simulink model "TST_AccPed_DrvDemDes"  (R2016b)
settings: Solver=FixedStepDiscrete  StartTime=0.0  StopTime=simTime  FixedStep=sampleTime  RelTol=1e-3
values from neighbouring files (symbols this model uses):
  testCase = 1    [initTST_AccPed_DrvDemDes_001.m]    (also in initTST_AccPed_DrvDemDes_002.m = 2; initTST_AccPed_DrvDemDes_003.m = 3; initTST_AccPed_DrvDemDes_004.m = 4; initTST_AccPed_DrvDemDes_005.m = 5)
libraries: simulink x61, UnitTest_Lib x54
(part 1 of 2)
settings Model: Creator=zhengjinyan  LastModifiedBy=zhengjinyan
settings DebuggingCC: SignalRangeChecking=error

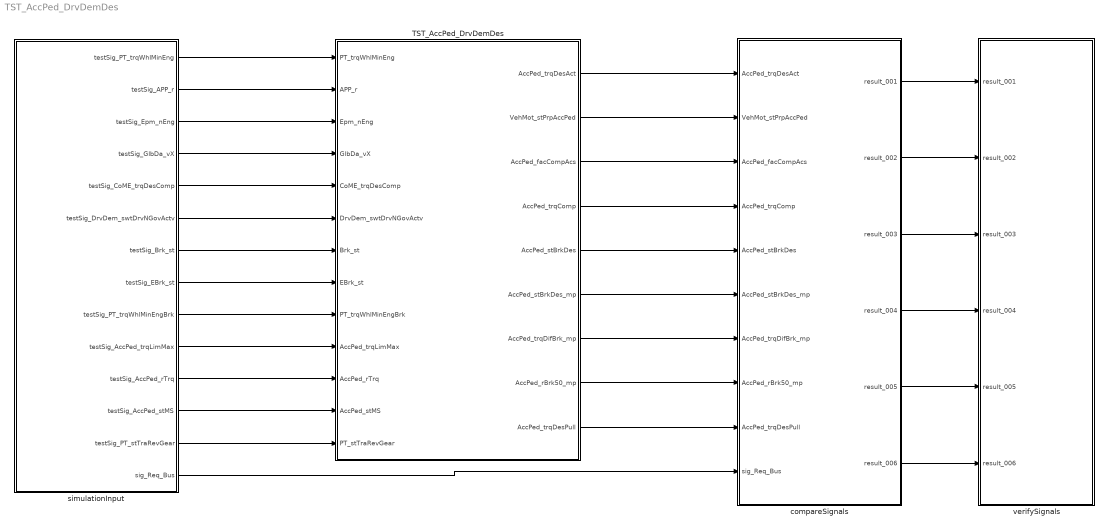
== system TST_AccPed_DrvDemDes ==
  TST_AccPed_DrvDemDes : Subsystem
  compareSignals : Subsystem
  simulationInput : Subsystem
  verifySignals : Subsystem
  wires:
  simulationInput/1(testSig_PT_trqWhlMinEng) -> TST_AccPed_DrvDemDes/1(PT_trqWhlMinEng)
  simulationInput/2(testSig_APP_r) -> TST_AccPed_DrvDemDes/2(APP_r)
  simulationInput/3(testSig_Epm_nEng) -> TST_AccPed_DrvDemDes/3(Epm_nEng)
  simulationInput/4(testSig_GlbDa_vX) -> TST_AccPed_DrvDemDes/4(GlbDa_vX)
  simulationInput/5(testSig_CoME_trqDesComp) -> TST_AccPed_DrvDemDes/5(CoME_trqDesComp)
  simulationInput/6(testSig_DrvDem_swtDrvNGovActv) -> TST_AccPed_DrvDemDes/6(DrvDem_swtDrvNGovActv)
  simulationInput/7(testSig_Brk_st) -> TST_AccPed_DrvDemDes/7(Brk_st)
  simulationInput/8(testSig_EBrk_st) -> TST_AccPed_DrvDemDes/8(EBrk_st)
  simulationInput/9(testSig_PT_trqWhlMinEngBrk) -> TST_AccPed_DrvDemDes/9(PT_trqWhlMinEngBrk)
  simulationInput/10(testSig_AccPed_trqLimMax) -> TST_AccPed_DrvDemDes/10(AccPed_trqLimMax)
  simulationInput/11(testSig_AccPed_rTrq) -> TST_AccPed_DrvDemDes/11(AccPed_rTrq)
  simulationInput/12(testSig_AccPed_stMS) -> TST_AccPed_DrvDemDes/12(AccPed_stMS)
  simulationInput/13(testSig_PT_stTraRevGear) -> TST_AccPed_DrvDemDes/13(PT_stTraRevGear)
  TST_AccPed_DrvDemDes/1(AccPed_trqDesAct) -> compareSignals/1(AccPed_trqDesAct)
  TST_AccPed_DrvDemDes/2(VehMot_stPrpAccPed) -> compareSignals/2(VehMot_stPrpAccPed)
  TST_AccPed_DrvDemDes/3(AccPed_facCompAcs) -> compareSignals/3(AccPed_facCompAcs)
  TST_AccPed_DrvDemDes/4(AccPed_trqComp) -> compareSignals/4(AccPed_trqComp)
  TST_AccPed_DrvDemDes/5(AccPed_stBrkDes) -> compareSignals/5(AccPed_stBrkDes)
  TST_AccPed_DrvDemDes/6(AccPed_stBrkDes_mp) -> compareSignals/6(AccPed_stBrkDes_mp)
  TST_AccPed_DrvDemDes/7(AccPed_trqDifBrk_mp) -> compareSignals/7(AccPed_trqDifBrk_mp)
  TST_AccPed_DrvDemDes/8(AccPed_rBrk50_mp) -> compareSignals/8(AccPed_rBrk50_mp)
  TST_AccPed_DrvDemDes/9(AccPed_trqDesPull) -> compareSignals/9(AccPed_trqDesPull)
  simulationInput/14(sig_Req_Bus) -> compareSignals/10(sig_Req_Bus)
  compareSignals/1(result_001) -> verifySignals/1(result_001)
  compareSignals/2(result_002) -> verifySignals/2(result_002)
  compareSignals/3(result_003) -> verifySignals/3(result_003)
  compareSignals/4(result_004) -> verifySignals/4(result_004)
  compareSignals/5(result_005) -> verifySignals/5(result_005)
  compareSignals/6(result_006) -> verifySignals/6(result_006)

== system TST_AccPed_DrvDemDes/TST_AccPed_DrvDemDes ==
  PT_trqWhlMinEng : Inport
  APP_r : Inport  Port=2
  Epm_nEng : Inport  Port=3
  GlbDa_vX : Inport  Port=4
  CoME_trqDesComp : Inport  Port=5
  DrvDem_swtDrvNGovActv : Inport  Port=6
  Brk_st : Inport  Port=7
  EBrk_st : Inport  Port=8
  PT_trqWhlMinEngBrk : Inport  Port=9
  AccPed_trqLimMax : Inport  Port=10
  AccPed_rTrq : Inport  Port=11
  AccPed_stMS : Inport  Port=12
  PT_stTraRevGear : Inport  Port=13
  AccPed_DrvDemDes : ModelReference  ModelNameDialog=AccPed_DrvDemDes  SimulationMode=Normal  ModelReferenceVersion=1.64  TriggerPortName=function  TriggerPortTriggerType=function-call  TriggerPortStatesWhenEnabling=held
  Function_Call : simulink/Ports & Subsystems/Function-Call Generator  sample_time=sampleTime  numberOfIterations=1
  AccPed_trqDesAct : Outport
  VehMot_stPrpAccPed : Outport  Port=2
  AccPed_facCompAcs : Outport  Port=3
  AccPed_trqComp : Outport  Port=4
  AccPed_stBrkDes : Outport  Port=5
  AccPed_stBrkDes_mp : Outport  Port=6
  AccPed_trqDifBrk_mp : Outport  Port=7
  AccPed_rBrk50_mp : Outport  Port=8
  AccPed_trqDesPull : Outport  Port=9
  wires:
  Function_Call/1 -> AccPed_DrvDemDes/Trigger
  PT_trqWhlMinEng/1 -> AccPed_DrvDemDes/1
  APP_r/1 -> AccPed_DrvDemDes/2
  Epm_nEng/1 -> AccPed_DrvDemDes/3
  GlbDa_vX/1 -> AccPed_DrvDemDes/4
  CoME_trqDesComp/1 -> AccPed_DrvDemDes/5
  DrvDem_swtDrvNGovActv/1 -> AccPed_DrvDemDes/6
  Brk_st/1 -> AccPed_DrvDemDes/7
  EBrk_st/1 -> AccPed_DrvDemDes/8
  PT_trqWhlMinEngBrk/1 -> AccPed_DrvDemDes/9
  AccPed_trqLimMax/1 -> AccPed_DrvDemDes/10
  AccPed_rTrq/1 -> AccPed_DrvDemDes/11
  AccPed_stMS/1 -> AccPed_DrvDemDes/12
  PT_stTraRevGear/1 -> AccPed_DrvDemDes/13
  AccPed_DrvDemDes/1 -> AccPed_trqDesAct/1
  AccPed_DrvDemDes/2 -> VehMot_stPrpAccPed/1
  AccPed_DrvDemDes/3 -> AccPed_facCompAcs/1
  AccPed_DrvDemDes/4 -> AccPed_trqComp/1
  AccPed_DrvDemDes/5 -> AccPed_stBrkDes/1
  AccPed_DrvDemDes/6 -> AccPed_stBrkDes_mp/1
  AccPed_DrvDemDes/7 -> AccPed_trqDifBrk_mp/1
  AccPed_DrvDemDes/8 -> AccPed_rBrk50_mp/1
  AccPed_DrvDemDes/9 -> AccPed_trqDesPull/1

== system TST_AccPed_DrvDemDes/compareSignals ==
  AccPed_trqDesAct : Inport
  VehMot_stPrpAccPed : Inport  Port=2
  AccPed_facCompAcs : Inport  Port=3
  AccPed_trqComp : Inport  Port=4
  AccPed_stBrkDes : Inport  Port=5
  AccPed_stBrkDes_mp : Inport  Port=6
  AccPed_trqDifBrk_mp : Inport  Port=7
  AccPed_rBrk50_mp : Inport  Port=8
  AccPed_trqDesPull : Inport  Port=9
  sig_Req_Bus : Inport  Port=10
  BC : BusCreator  Inputs=9
  CTC_001 : simulink/Logic and Bit Operations/Compare To Constant  relop===  const=1  OutDataTypeStr=boolean
  CTC_002 : simulink/Logic and Bit Operations/Compare To Constant  relop===  const=2  OutDataTypeStr=boolean
  CTC_003 : simulink/Logic and Bit Operations/Compare To Constant  relop===  const=3  OutDataTypeStr=boolean
  CTC_004 : simulink/Logic and Bit Operations/Compare To Constant  relop===  const=4  OutDataTypeStr=boolean
  CTC_005 : simulink/Logic and Bit Operations/Compare To Constant  relop===  const=5  OutDataTypeStr=boolean
  CTC_006 : simulink/Logic and Bit Operations/Compare To Constant  relop===  const=6  OutDataTypeStr=boolean
  Requirement_001 : Subsystem
  Requirement_002 : Subsystem
  Requirement_003 : Subsystem
  Requirement_004 : Subsystem
  Requirement_005 : Subsystem
  Requirement_006 : Subsystem
  TC_001 : Constant  Value=testCase
  TC_002 : Constant  Value=testCase
  TC_003 : Constant  Value=testCase
  TC_004 : Constant  Value=testCase
  TC_005 : Constant  Value=testCase
  TC_006 : Constant  Value=testCase
  result_001 : Outport
  result_002 : Outport  Port=2
  result_003 : Outport  Port=3
  result_004 : Outport  Port=4
  result_005 : Outport  Port=5
  result_006 : Outport  Port=6
  wires:
  AccPed_trqDesAct/1 -> BC/1  "AccPed_trqDesAct"
  VehMot_stPrpAccPed/1 -> BC/2  "VehMot_stPrpAccPed"
  AccPed_facCompAcs/1 -> BC/3  "AccPed_facCompAcs"
  AccPed_trqComp/1 -> BC/4  "AccPed_trqComp"
  AccPed_stBrkDes/1 -> BC/5  "AccPed_stBrkDes"
  AccPed_stBrkDes_mp/1 -> BC/6  "AccPed_stBrkDes_mp"
  AccPed_trqDifBrk_mp/1 -> BC/7  "AccPed_trqDifBrk_mp"
  AccPed_rBrk50_mp/1 -> BC/8  "AccPed_rBrk50_mp"
  AccPed_trqDesPull/1 -> BC/9  "AccPed_trqDesPull"
  TC_001/1 -> CTC_001/1
  CTC_001/1 -> Requirement_001/Enable
  sig_Req_Bus/1 -> Requirement_001/2(sig_Req_Bus), Requirement_002/2(sig_Req_Bus), Requirement_003/2(sig_Req_Bus), Requirement_004/2(sig_Req_Bus), Requirement_005/2(sig_Req_Bus), Requirement_006/2(sig_Req_Bus)
  BC/1 -> Requirement_001/1(sig_Result_Bus), Requirement_002/1(sig_Result_Bus), Requirement_003/1(sig_Result_Bus), Requirement_004/1(sig_Result_Bus), Requirement_005/1(sig_Result_Bus), Requirement_006/1(sig_Result_Bus)
  Requirement_001/1(result) -> result_001/1
  TC_002/1 -> CTC_002/1
  CTC_002/1 -> Requirement_002/Enable
  Requirement_002/1(result) -> result_002/1
  TC_003/1 -> CTC_003/1
  CTC_003/1 -> Requirement_003/Enable
  Requirement_003/1(result) -> result_003/1
  TC_004/1 -> CTC_004/1
  CTC_004/1 -> Requirement_004/Enable
  Requirement_004/1(result) -> result_004/1
  TC_005/1 -> CTC_005/1
  CTC_005/1 -> Requirement_005/Enable
  Requirement_005/1(result) -> result_005/1
  TC_006/1 -> CTC_006/1
  CTC_006/1 -> Requirement_006/Enable
  Requirement_006/1(result) -> result_006/1

== system TST_AccPed_DrvDemDes/simulationInput ==
  BS : BusSelector  OutputSignals=testSig_PT_trqWhlMinEng,testSig_APP_r,testSig_Epm_nEng,testSig_GlbDa_vX,testSig_CoME_trqDesComp,testSig_DrvDem_swtDrvNGovActv,testSig_Brk_st,testSig_EBrk_st,testSig_PT_trqWhlMinEngBrk,testSig_AccPed_trqLimMax,testSig_AccPed_rTrq,testSig_AccPed_stMS,testSig_PT_stTraRevGear
  MPSw : MultiPortSwitch  Inputs=6  SaturateOnIntegerOverflow=on  InputSameDT=on
  TestCase : Constant  Value=testCase
  testSignals_R001 : Subsystem
  testSignals_R002 : Subsystem
  testSignals_R003 : Subsystem
  testSignals_R004 : Subsystem
  testSignals_R005 : Subsystem
  testSignals_R006 : Subsystem
  testSig_PT_trqWhlMinEng : Outport
  testSig_APP_r : Outport  Port=2
  testSig_Epm_nEng : Outport  Port=3
  testSig_GlbDa_vX : Outport  Port=4
  testSig_CoME_trqDesComp : Outport  Port=5
  testSig_DrvDem_swtDrvNGovActv : Outport  Port=6
  testSig_Brk_st : Outport  Port=7
  testSig_EBrk_st : Outport  Port=8
  testSig_PT_trqWhlMinEngBrk : Outport  Port=9
  testSig_AccPed_trqLimMax : Outport  Port=10
  testSig_AccPed_rTrq : Outport  Port=11
  testSig_AccPed_stMS : Outport  Port=12
  testSig_PT_stTraRevGear : Outport  Port=13
  sig_Req_Bus : Outport  Port=14
  wires:
  BS/1 -> testSig_PT_trqWhlMinEng/1  "<testSig_PT_trqWhlMinEng>"
  BS/2 -> testSig_APP_r/1  "<testSig_APP_r>"
  BS/3 -> testSig_Epm_nEng/1  "<testSig_Epm_nEng>"
  BS/4 -> testSig_GlbDa_vX/1  "<testSig_GlbDa_vX>"
  BS/5 -> testSig_CoME_trqDesComp/1  "<testSig_CoME_trqDesComp>"
  BS/6 -> testSig_DrvDem_swtDrvNGovActv/1  "<testSig_DrvDem_swtDrvNGovActv>"
  BS/7 -> testSig_Brk_st/1  "<testSig_Brk_st>"
  BS/8 -> testSig_EBrk_st/1  "<testSig_EBrk_st>"
  BS/9 -> testSig_PT_trqWhlMinEngBrk/1  "<testSig_PT_trqWhlMinEngBrk>"
  BS/10 -> testSig_AccPed_trqLimMax/1  "<testSig_AccPed_trqLimMax>"
  BS/11 -> testSig_AccPed_rTrq/1  "<testSig_AccPed_rTrq>"
  BS/12 -> testSig_AccPed_stMS/1  "<testSig_AccPed_stMS>"
  BS/13 -> testSig_PT_stTraRevGear/1  "<testSig_PT_stTraRevGear>"
  MPSw/1 -> BS/1, sig_Req_Bus/1
  TestCase/1 -> MPSw/1
  testSignals_R001/1(testSignals) -> MPSw/2
  testSignals_R002/1(testSignals) -> MPSw/3
  testSignals_R003/1(testSignals) -> MPSw/4
  testSignals_R004/1(testSignals) -> MPSw/5
  testSignals_R005/1(testSignals) -> MPSw/6
  testSignals_R006/1(testSignals) -> MPSw/7

== system TST_AccPed_DrvDemDes/verifySignals ==
  result_001 : Inport
  result_002 : Inport  Port=2
  result_003 : Inport  Port=3
  result_004 : Inport  Port=4
  result_005 : Inport  Port=5
  result_006 : Inport  Port=6
  Assertion_001 : Assertion  Enabled=off
  Assertion_002 : Assertion  Enabled=off
  Assertion_003 : Assertion  Enabled=off
  Assertion_004 : Assertion  Enabled=off
  Assertion_005 : Assertion  Enabled=off
  Assertion_006 : Assertion  Enabled=off
  wires:
  result_001/1 -> Assertion_001/1
  result_002/1 -> Assertion_002/1
  result_003/1 -> Assertion_003/1
  result_004/1 -> Assertion_004/1
  result_005/1 -> Assertion_005/1
  result_006/1 -> Assertion_006/1

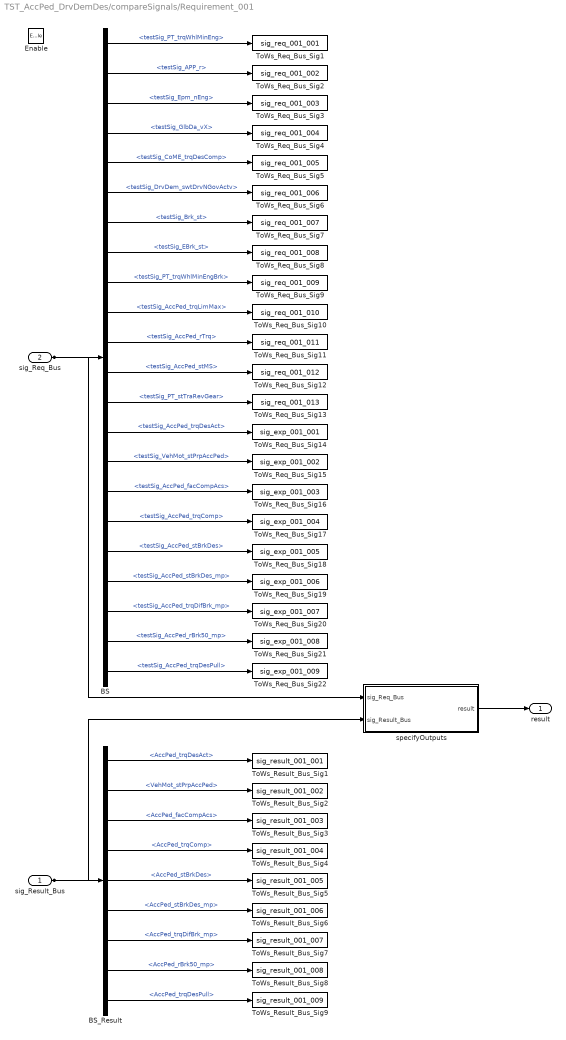
== system TST_AccPed_DrvDemDes/compareSignals/Requirement_001 ==
  sig_Result_Bus : Inport
  sig_Req_Bus : Inport  Port=2
  Enable : EnablePort
  BS : BusSelector  OutputSignals=testSig_PT_trqWhlMinEng,testSig_APP_r,testSig_Epm_nEng,testSig_GlbDa_vX,testSig_CoME_trqDesComp,testSig_DrvDem_swtDrvNGovActv,testSig_Brk_st,testSig_EBrk_st,testSig_PT_trqWhlMinEngBrk,testSig_AccPed_trqLimMax,testSig_AccPed_rTrq,testSig_AccPed_stMS,testSig_PT_stTraRevGear,testSig_AccPed_trqDesAct,testSig_VehMot_stPrpAccPed,testSig_AccPed_facCompAcs,testSig_AccPed_trqComp,testSig_AccPed_stBrkDes,testSig_AccPed_stBrkDes_mp,testSig_AccPed_trqDifBrk_mp,testSig_AccPed_rBrk50_mp,testSig_AccPed_trqDesPull
  BS_Result : BusSelector  OutputSignals=AccPed_trqDesAct,VehMot_stPrpAccPed,AccPed_facCompAcs,AccPed_trqComp,AccPed_stBrkDes,AccPed_stBrkDes_mp,AccPed_trqDifBrk_mp,AccPed_rBrk50_mp,AccPed_trqDesPull
  ToWs_Req_Bus_Sig1 : ToWorkspace  VariableName=sig_req_001_001  SaveFormat=Structure With Time
  ToWs_Req_Bus_Sig10 : ToWorkspace  VariableName=sig_req_001_010  SaveFormat=Structure With Time
  ToWs_Req_Bus_Sig11 : ToWorkspace  VariableName=sig_req_001_011  SaveFormat=Structure With Time
  ToWs_Req_Bus_Sig12 : ToWorkspace  VariableName=sig_req_001_012  SaveFormat=Structure With Time
  ToWs_Req_Bus_Sig13 : ToWorkspace  VariableName=sig_req_001_013  SaveFormat=Structure With Time
  ToWs_Req_Bus_Sig14 : ToWorkspace  VariableName=sig_exp_001_001  SaveFormat=Structure With Time
  ToWs_Req_Bus_Sig15 : ToWorkspace  VariableName=sig_exp_001_002  SaveFormat=Structure With Time
  ToWs_Req_Bus_Sig16 : ToWorkspace  VariableName=sig_exp_001_003  SaveFormat=Structure With Time
  ToWs_Req_Bus_Sig17 : ToWorkspace  VariableName=sig_exp_001_004  SaveFormat=Structure With Time
  ToWs_Req_Bus_Sig18 : ToWorkspace  VariableName=sig_exp_001_005  SaveFormat=Structure With Time
  ToWs_Req_Bus_Sig19 : ToWorkspace  VariableName=sig_exp_001_006  SaveFormat=Structure With Time
  ToWs_Req_Bus_Sig2 : ToWorkspace  VariableName=sig_req_001_002  SaveFormat=Structure With Time
  ToWs_Req_Bus_Sig20 : ToWorkspace  VariableName=sig_exp_001_007  SaveFormat=Structure With Time
  ToWs_Req_Bus_Sig21 : ToWorkspace  VariableName=sig_exp_001_008  SaveFormat=Structure With Time
  ToWs_Req_Bus_Sig22 : ToWorkspace  VariableName=sig_exp_001_009  SaveFormat=Structure With Time
  ToWs_Req_Bus_Sig3 : ToWorkspace  VariableName=sig_req_001_003  SaveFormat=Structure With Time
  ToWs_Req_Bus_Sig4 : ToWorkspace  VariableName=sig_req_001_004  SaveFormat=Structure With Time
  ToWs_Req_Bus_Sig5 : ToWorkspace  VariableName=sig_req_001_005  SaveFormat=Structure With Time
  ToWs_Req_Bus_Sig6 : ToWorkspace  VariableName=sig_req_001_006  SaveFormat=Structure With Time
  ToWs_Req_Bus_Sig7 : ToWorkspace  VariableName=sig_req_001_007  SaveFormat=Structure With Time
  ToWs_Req_Bus_Sig8 : ToWorkspace  VariableName=sig_req_001_008  SaveFormat=Structure With Time
  ToWs_Req_Bus_Sig9 : ToWorkspace  VariableName=sig_req_001_009  SaveFormat=Structure With Time
  ToWs_Result_Bus_Sig1 : ToWorkspace  VariableName=sig_result_001_001  SaveFormat=Structure With Time
  ToWs_Result_Bus_Sig2 : ToWorkspace  VariableName=sig_result_001_002  SaveFormat=Structure With Time
  ToWs_Result_Bus_Sig3 : ToWorkspace  VariableName=sig_result_001_003  SaveFormat=Structure With Time
  ToWs_Result_Bus_Sig4 : ToWorkspace  VariableName=sig_result_001_004  SaveFormat=Structure With Time
  ToWs_Result_Bus_Sig5 : ToWorkspace  VariableName=sig_result_001_005  SaveFormat=Structure With Time
  ToWs_Result_Bus_Sig6 : ToWorkspace  VariableName=sig_result_001_006  SaveFormat=Structure With Time
  ToWs_Result_Bus_Sig7 : ToWorkspace  VariableName=sig_result_001_007  SaveFormat=Structure With Time
  ToWs_Result_Bus_Sig8 : ToWorkspace  VariableName=sig_result_001_008  SaveFormat=Structure With Time
  ToWs_Result_Bus_Sig9 : ToWorkspace  VariableName=sig_result_001_009  SaveFormat=Structure With Time
  specifyOutputs : Subsystem
  result : Outport
  wires:
  sig_Req_Bus/1 -> BS/1, specifyOutputs/1(sig_Req_Bus)
  BS/1 -> ToWs_Req_Bus_Sig1/1  "<testSig_PT_trqWhlMinEng>"
  BS/2 -> ToWs_Req_Bus_Sig2/1  "<testSig_APP_r>"
  BS/3 -> ToWs_Req_Bus_Sig3/1  "<testSig_Epm_nEng>"
  BS/4 -> ToWs_Req_Bus_Sig4/1  "<testSig_GlbDa_vX>"
  BS/5 -> ToWs_Req_Bus_Sig5/1  "<testSig_CoME_trqDesComp>"
  BS/6 -> ToWs_Req_Bus_Sig6/1  "<testSig_DrvDem_swtDrvNGovActv>"
  BS/7 -> ToWs_Req_Bus_Sig7/1  "<testSig_Brk_st>"
  BS/8 -> ToWs_Req_Bus_Sig8/1  "<testSig_EBrk_st>"
  BS/9 -> ToWs_Req_Bus_Sig9/1  "<testSig_PT_trqWhlMinEngBrk>"
  BS/10 -> ToWs_Req_Bus_Sig10/1  "<testSig_AccPed_trqLimMax>"
  BS/11 -> ToWs_Req_Bus_Sig11/1  "<testSig_AccPed_rTrq>"
  BS/12 -> ToWs_Req_Bus_Sig12/1  "<testSig_AccPed_stMS>"
  BS/13 -> ToWs_Req_Bus_Sig13/1  "<testSig_PT_stTraRevGear>"
  BS/14 -> ToWs_Req_Bus_Sig14/1  "<testSig_AccPed_trqDesAct>"
  BS/15 -> ToWs_Req_Bus_Sig15/1  "<testSig_VehMot_stPrpAccPed>"
  BS/16 -> ToWs_Req_Bus_Sig16/1  "<testSig_AccPed_facCompAcs>"
  BS/17 -> ToWs_Req_Bus_Sig17/1  "<testSig_AccPed_trqComp>"
  BS/18 -> ToWs_Req_Bus_Sig18/1  "<testSig_AccPed_stBrkDes>"
  BS/19 -> ToWs_Req_Bus_Sig19/1  "<testSig_AccPed_stBrkDes_mp>"
  BS/20 -> ToWs_Req_Bus_Sig20/1  "<testSig_AccPed_trqDifBrk_mp>"
  BS/21 -> ToWs_Req_Bus_Sig21/1  "<testSig_AccPed_rBrk50_mp>"
  BS/22 -> ToWs_Req_Bus_Sig22/1  "<testSig_AccPed_trqDesPull>"
  sig_Result_Bus/1 -> BS_Result/1, specifyOutputs/2(sig_Result_Bus)
  BS_Result/1 -> ToWs_Result_Bus_Sig1/1  "<AccPed_trqDesAct>"
  BS_Result/2 -> ToWs_Result_Bus_Sig2/1  "<VehMot_stPrpAccPed>"
  BS_Result/3 -> ToWs_Result_Bus_Sig3/1  "<AccPed_facCompAcs>"
  BS_Result/4 -> ToWs_Result_Bus_Sig4/1  "<AccPed_trqComp>"
  BS_Result/5 -> ToWs_Result_Bus_Sig5/1  "<AccPed_stBrkDes>"
  BS_Result/6 -> ToWs_Result_Bus_Sig6/1  "<AccPed_stBrkDes_mp>"
  BS_Result/7 -> ToWs_Result_Bus_Sig7/1  "<AccPed_trqDifBrk_mp>"
  BS_Result/8 -> ToWs_Result_Bus_Sig8/1  "<AccPed_rBrk50_mp>"
  BS_Result/9 -> ToWs_Result_Bus_Sig9/1  "<AccPed_trqDesPull>"
  specifyOutputs/1(result) -> result/1

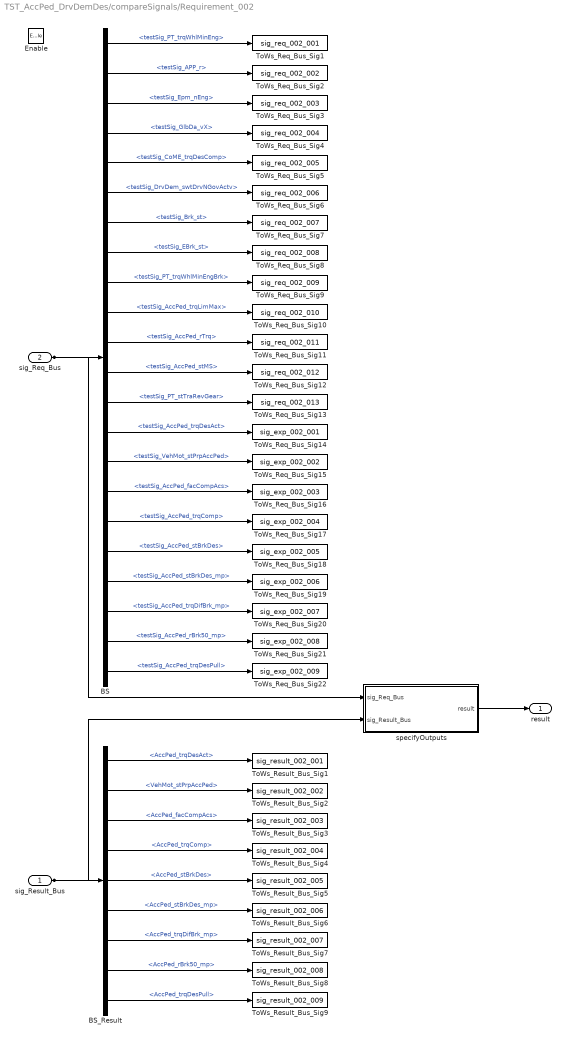
== system TST_AccPed_DrvDemDes/compareSignals/Requirement_002 ==
  sig_Result_Bus : Inport
  sig_Req_Bus : Inport  Port=2
  Enable : EnablePort
  BS : BusSelector  OutputSignals=testSig_PT_trqWhlMinEng,testSig_APP_r,testSig_Epm_nEng,testSig_GlbDa_vX,testSig_CoME_trqDesComp,testSig_DrvDem_swtDrvNGovActv,testSig_Brk_st,testSig_EBrk_st,testSig_PT_trqWhlMinEngBrk,testSig_AccPed_trqLimMax,testSig_AccPed_rTrq,testSig_AccPed_stMS,testSig_PT_stTraRevGear,testSig_AccPed_trqDesAct,testSig_VehMot_stPrpAccPed,testSig_AccPed_facCompAcs,testSig_AccPed_trqComp,testSig_AccPed_stBrkDes,testSig_AccPed_stBrkDes_mp,testSig_AccPed_trqDifBrk_mp,testSig_AccPed_rBrk50_mp,testSig_AccPed_trqDesPull
  BS_Result : BusSelector  OutputSignals=AccPed_trqDesAct,VehMot_stPrpAccPed,AccPed_facCompAcs,AccPed_trqComp,AccPed_stBrkDes,AccPed_stBrkDes_mp,AccPed_trqDifBrk_mp,AccPed_rBrk50_mp,AccPed_trqDesPull
  ToWs_Req_Bus_Sig1 : ToWorkspace  VariableName=sig_req_002_001  SaveFormat=Structure With Time
  ToWs_Req_Bus_Sig10 : ToWorkspace  VariableName=sig_req_002_010  SaveFormat=Structure With Time
  ToWs_Req_Bus_Sig11 : ToWorkspace  VariableName=sig_req_002_011  SaveFormat=Structure With Time
  ToWs_Req_Bus_Sig12 : ToWorkspace  VariableName=sig_req_002_012  SaveFormat=Structure With Time
  ToWs_Req_Bus_Sig13 : ToWorkspace  VariableName=sig_req_002_013  SaveFormat=Structure With Time
  ToWs_Req_Bus_Sig14 : ToWorkspace  VariableName=sig_exp_002_001  SaveFormat=Structure With Time
  ToWs_Req_Bus_Sig15 : ToWorkspace  VariableName=sig_exp_002_002  SaveFormat=Structure With Time
  ToWs_Req_Bus_Sig16 : ToWorkspace  VariableName=sig_exp_002_003  SaveFormat=Structure With Time
  ToWs_Req_Bus_Sig17 : ToWorkspace  VariableName=sig_exp_002_004  SaveFormat=Structure With Time
  ToWs_Req_Bus_Sig18 : ToWorkspace  VariableName=sig_exp_002_005  SaveFormat=Structure With Time
  ToWs_Req_Bus_Sig19 : ToWorkspace  VariableName=sig_exp_002_006  SaveFormat=Structure With Time
  ToWs_Req_Bus_Sig2 : ToWorkspace  VariableName=sig_req_002_002  SaveFormat=Structure With Time
  ToWs_Req_Bus_Sig20 : ToWorkspace  VariableName=sig_exp_002_007  SaveFormat=Structure With Time
  ToWs_Req_Bus_Sig21 : ToWorkspace  VariableName=sig_exp_002_008  SaveFormat=Structure With Time
  ToWs_Req_Bus_Sig22 : ToWorkspace  VariableName=sig_exp_002_009  SaveFormat=Structure With Time
  ToWs_Req_Bus_Sig3 : ToWorkspace  VariableName=sig_req_002_003  SaveFormat=Structure With Time
  ToWs_Req_Bus_Sig4 : ToWorkspace  VariableName=sig_req_002_004  SaveFormat=Structure With Time
  ToWs_Req_Bus_Sig5 : ToWorkspace  VariableName=sig_req_002_005  SaveFormat=Structure With Time
  ToWs_Req_Bus_Sig6 : ToWorkspace  VariableName=sig_req_002_006  SaveFormat=Structure With Time
  ToWs_Req_Bus_Sig7 : ToWorkspace  VariableName=sig_req_002_007  SaveFormat=Structure With Time
  ToWs_Req_Bus_Sig8 : ToWorkspace  VariableName=sig_req_002_008  SaveFormat=Structure With Time
  ToWs_Req_Bus_Sig9 : ToWorkspace  VariableName=sig_req_002_009  SaveFormat=Structure With Time
  ToWs_Result_Bus_Sig1 : ToWorkspace  VariableName=sig_result_002_001  SaveFormat=Structure With Time
  ToWs_Result_Bus_Sig2 : ToWorkspace  VariableName=sig_result_002_002  SaveFormat=Structure With Time
  ToWs_Result_Bus_Sig3 : ToWorkspace  VariableName=sig_result_002_003  SaveFormat=Structure With Time
  ToWs_Result_Bus_Sig4 : ToWorkspace  VariableName=sig_result_002_004  SaveFormat=Structure With Time
  ToWs_Result_Bus_Sig5 : ToWorkspace  VariableName=sig_result_002_005  SaveFormat=Structure With Time
  ToWs_Result_Bus_Sig6 : ToWorkspace  VariableName=sig_result_002_006  SaveFormat=Structure With Time
  ToWs_Result_Bus_Sig7 : ToWorkspace  VariableName=sig_result_002_007  SaveFormat=Structure With Time
  ToWs_Result_Bus_Sig8 : ToWorkspace  VariableName=sig_result_002_008  SaveFormat=Structure With Time
  ToWs_Result_Bus_Sig9 : ToWorkspace  VariableName=sig_result_002_009  SaveFormat=Structure With Time
  specifyOutputs : Subsystem
  result : Outport
  wires:
  sig_Req_Bus/1 -> BS/1, specifyOutputs/1(sig_Req_Bus)
  BS/1 -> ToWs_Req_Bus_Sig1/1  "<testSig_PT_trqWhlMinEng>"
  BS/2 -> ToWs_Req_Bus_Sig2/1  "<testSig_APP_r>"
  BS/3 -> ToWs_Req_Bus_Sig3/1  "<testSig_Epm_nEng>"
  BS/4 -> ToWs_Req_Bus_Sig4/1  "<testSig_GlbDa_vX>"
  BS/5 -> ToWs_Req_Bus_Sig5/1  "<testSig_CoME_trqDesComp>"
  BS/6 -> ToWs_Req_Bus_Sig6/1  "<testSig_DrvDem_swtDrvNGovActv>"
  BS/7 -> ToWs_Req_Bus_Sig7/1  "<testSig_Brk_st>"
  BS/8 -> ToWs_Req_Bus_Sig8/1  "<testSig_EBrk_st>"
  BS/9 -> ToWs_Req_Bus_Sig9/1  "<testSig_PT_trqWhlMinEngBrk>"
  BS/10 -> ToWs_Req_Bus_Sig10/1  "<testSig_AccPed_trqLimMax>"
  BS/11 -> ToWs_Req_Bus_Sig11/1  "<testSig_AccPed_rTrq>"
  BS/12 -> ToWs_Req_Bus_Sig12/1  "<testSig_AccPed_stMS>"
  BS/13 -> ToWs_Req_Bus_Sig13/1  "<testSig_PT_stTraRevGear>"
  BS/14 -> ToWs_Req_Bus_Sig14/1  "<testSig_AccPed_trqDesAct>"
  BS/15 -> ToWs_Req_Bus_Sig15/1  "<testSig_VehMot_stPrpAccPed>"
  BS/16 -> ToWs_Req_Bus_Sig16/1  "<testSig_AccPed_facCompAcs>"
  BS/17 -> ToWs_Req_Bus_Sig17/1  "<testSig_AccPed_trqComp>"
  BS/18 -> ToWs_Req_Bus_Sig18/1  "<testSig_AccPed_stBrkDes>"
  BS/19 -> ToWs_Req_Bus_Sig19/1  "<testSig_AccPed_stBrkDes_mp>"
  BS/20 -> ToWs_Req_Bus_Sig20/1  "<testSig_AccPed_trqDifBrk_mp>"
  BS/21 -> ToWs_Req_Bus_Sig21/1  "<testSig_AccPed_rBrk50_mp>"
  BS/22 -> ToWs_Req_Bus_Sig22/1  "<testSig_AccPed_trqDesPull>"
  sig_Result_Bus/1 -> BS_Result/1, specifyOutputs/2(sig_Result_Bus)
  BS_Result/1 -> ToWs_Result_Bus_Sig1/1  "<AccPed_trqDesAct>"
  BS_Result/2 -> ToWs_Result_Bus_Sig2/1  "<VehMot_stPrpAccPed>"
  BS_Result/3 -> ToWs_Result_Bus_Sig3/1  "<AccPed_facCompAcs>"
  BS_Result/4 -> ToWs_Result_Bus_Sig4/1  "<AccPed_trqComp>"
  BS_Result/5 -> ToWs_Result_Bus_Sig5/1  "<AccPed_stBrkDes>"
  BS_Result/6 -> ToWs_Result_Bus_Sig6/1  "<AccPed_stBrkDes_mp>"
  BS_Result/7 -> ToWs_Result_Bus_Sig7/1  "<AccPed_trqDifBrk_mp>"
  BS_Result/8 -> ToWs_Result_Bus_Sig8/1  "<AccPed_rBrk50_mp>"
  BS_Result/9 -> ToWs_Result_Bus_Sig9/1  "<AccPed_trqDesPull>"
  specifyOutputs/1(result) -> result/1

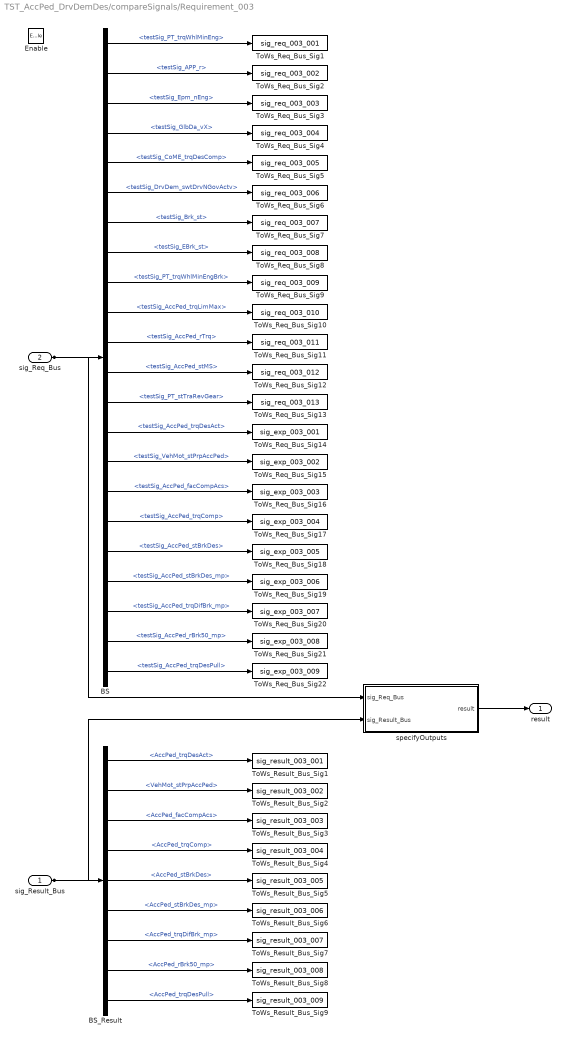
== system TST_AccPed_DrvDemDes/compareSignals/Requirement_003 ==
  sig_Result_Bus : Inport
  sig_Req_Bus : Inport  Port=2
  Enable : EnablePort
  BS : BusSelector  OutputSignals=testSig_PT_trqWhlMinEng,testSig_APP_r,testSig_Epm_nEng,testSig_GlbDa_vX,testSig_CoME_trqDesComp,testSig_DrvDem_swtDrvNGovActv,testSig_Brk_st,testSig_EBrk_st,testSig_PT_trqWhlMinEngBrk,testSig_AccPed_trqLimMax,testSig_AccPed_rTrq,testSig_AccPed_stMS,testSig_PT_stTraRevGear,testSig_AccPed_trqDesAct,testSig_VehMot_stPrpAccPed,testSig_AccPed_facCompAcs,testSig_AccPed_trqComp,testSig_AccPed_stBrkDes,testSig_AccPed_stBrkDes_mp,testSig_AccPed_trqDifBrk_mp,testSig_AccPed_rBrk50_mp,testSig_AccPed_trqDesPull
  BS_Result : BusSelector  OutputSignals=AccPed_trqDesAct,VehMot_stPrpAccPed,AccPed_facCompAcs,AccPed_trqComp,AccPed_stBrkDes,AccPed_stBrkDes_mp,AccPed_trqDifBrk_mp,AccPed_rBrk50_mp,AccPed_trqDesPull
  ToWs_Req_Bus_Sig1 : ToWorkspace  VariableName=sig_req_003_001  SaveFormat=Structure With Time
  ToWs_Req_Bus_Sig10 : ToWorkspace  VariableName=sig_req_003_010  SaveFormat=Structure With Time
  ToWs_Req_Bus_Sig11 : ToWorkspace  VariableName=sig_req_003_011  SaveFormat=Structure With Time
  ToWs_Req_Bus_Sig12 : ToWorkspace  VariableName=sig_req_003_012  SaveFormat=Structure With Time
  ToWs_Req_Bus_Sig13 : ToWorkspace  VariableName=sig_req_003_013  SaveFormat=Structure With Time
  ToWs_Req_Bus_Sig14 : ToWorkspace  VariableName=sig_exp_003_001  SaveFormat=Structure With Time
  ToWs_Req_Bus_Sig15 : ToWorkspace  VariableName=sig_exp_003_002  SaveFormat=Structure With Time
  ToWs_Req_Bus_Sig16 : ToWorkspace  VariableName=sig_exp_003_003  SaveFormat=Structure With Time
  ToWs_Req_Bus_Sig17 : ToWorkspace  VariableName=sig_exp_003_004  SaveFormat=Structure With Time
  ToWs_Req_Bus_Sig18 : ToWorkspace  VariableName=sig_exp_003_005  SaveFormat=Structure With Time
  ToWs_Req_Bus_Sig19 : ToWorkspace  VariableName=sig_exp_003_006  SaveFormat=Structure With Time
  ToWs_Req_Bus_Sig2 : ToWorkspace  VariableName=sig_req_003_002  SaveFormat=Structure With Time
  ToWs_Req_Bus_Sig20 : ToWorkspace  VariableName=sig_exp_003_007  SaveFormat=Structure With Time
  ToWs_Req_Bus_Sig21 : ToWorkspace  VariableName=sig_exp_003_008  SaveFormat=Structure With Time
  ToWs_Req_Bus_Sig22 : ToWorkspace  VariableName=sig_exp_003_009  SaveFormat=Structure With Time
  ToWs_Req_Bus_Sig3 : ToWorkspace  VariableName=sig_req_003_003  SaveFormat=Structure With Time
  ToWs_Req_Bus_Sig4 : ToWorkspace  VariableName=sig_req_003_004  SaveFormat=Structure With Time
  ToWs_Req_Bus_Sig5 : ToWorkspace  VariableName=sig_req_003_005  SaveFormat=Structure With Time
  ToWs_Req_Bus_Sig6 : ToWorkspace  VariableName=sig_req_003_006  SaveFormat=Structure With Time
  ToWs_Req_Bus_Sig7 : ToWorkspace  VariableName=sig_req_003_007  SaveFormat=Structure With Time
  ToWs_Req_Bus_Sig8 : ToWorkspace  VariableName=sig_req_003_008  SaveFormat=Structure With Time
  ToWs_Req_Bus_Sig9 : ToWorkspace  VariableName=sig_req_003_009  SaveFormat=Structure With Time
  ToWs_Result_Bus_Sig1 : ToWorkspace  VariableName=sig_result_003_001  SaveFormat=Structure With Time
  ToWs_Result_Bus_Sig2 : ToWorkspace  VariableName=sig_result_003_002  SaveFormat=Structure With Time
  ToWs_Result_Bus_Sig3 : ToWorkspace  VariableName=sig_result_003_003  SaveFormat=Structure With Time
  ToWs_Result_Bus_Sig4 : ToWorkspace  VariableName=sig_result_003_004  SaveFormat=Structure With Time
  ToWs_Result_Bus_Sig5 : ToWorkspace  VariableName=sig_result_003_005  SaveFormat=Structure With Time
  ToWs_Result_Bus_Sig6 : ToWorkspace  VariableName=sig_result_003_006  SaveFormat=Structure With Time
  ToWs_Result_Bus_Sig7 : ToWorkspace  VariableName=sig_result_003_007  SaveFormat=Structure With Time
  ToWs_Result_Bus_Sig8 : ToWorkspace  VariableName=sig_result_003_008  SaveFormat=Structure With Time
  ToWs_Result_Bus_Sig9 : ToWorkspace  VariableName=sig_result_003_009  SaveFormat=Structure With Time
  specifyOutputs : Subsystem
  result : Outport
  wires:
  sig_Req_Bus/1 -> BS/1, specifyOutputs/1(sig_Req_Bus)
  BS/1 -> ToWs_Req_Bus_Sig1/1  "<testSig_PT_trqWhlMinEng>"
  BS/2 -> ToWs_Req_Bus_Sig2/1  "<testSig_APP_r>"
  BS/3 -> ToWs_Req_Bus_Sig3/1  "<testSig_Epm_nEng>"
  BS/4 -> ToWs_Req_Bus_Sig4/1  "<testSig_GlbDa_vX>"
  BS/5 -> ToWs_Req_Bus_Sig5/1  "<testSig_CoME_trqDesComp>"
  BS/6 -> ToWs_Req_Bus_Sig6/1  "<testSig_DrvDem_swtDrvNGovActv>"
  BS/7 -> ToWs_Req_Bus_Sig7/1  "<testSig_Brk_st>"
  BS/8 -> ToWs_Req_Bus_Sig8/1  "<testSig_EBrk_st>"
  BS/9 -> ToWs_Req_Bus_Sig9/1  "<testSig_PT_trqWhlMinEngBrk>"
  BS/10 -> ToWs_Req_Bus_Sig10/1  "<testSig_AccPed_trqLimMax>"
  BS/11 -> ToWs_Req_Bus_Sig11/1  "<testSig_AccPed_rTrq>"
  BS/12 -> ToWs_Req_Bus_Sig12/1  "<testSig_AccPed_stMS>"
  BS/13 -> ToWs_Req_Bus_Sig13/1  "<testSig_PT_stTraRevGear>"
  BS/14 -> ToWs_Req_Bus_Sig14/1  "<testSig_AccPed_trqDesAct>"
  BS/15 -> ToWs_Req_Bus_Sig15/1  "<testSig_VehMot_stPrpAccPed>"
  BS/16 -> ToWs_Req_Bus_Sig16/1  "<testSig_AccPed_facCompAcs>"
  BS/17 -> ToWs_Req_Bus_Sig17/1  "<testSig_AccPed_trqComp>"
  BS/18 -> ToWs_Req_Bus_Sig18/1  "<testSig_AccPed_stBrkDes>"
  BS/19 -> ToWs_Req_Bus_Sig19/1  "<testSig_AccPed_stBrkDes_mp>"
  BS/20 -> ToWs_Req_Bus_Sig20/1  "<testSig_AccPed_trqDifBrk_mp>"
  BS/21 -> ToWs_Req_Bus_Sig21/1  "<testSig_AccPed_rBrk50_mp>"
  BS/22 -> ToWs_Req_Bus_Sig22/1  "<testSig_AccPed_trqDesPull>"
  sig_Result_Bus/1 -> BS_Result/1, specifyOutputs/2(sig_Result_Bus)
  BS_Result/1 -> ToWs_Result_Bus_Sig1/1  "<AccPed_trqDesAct>"
  BS_Result/2 -> ToWs_Result_Bus_Sig2/1  "<VehMot_stPrpAccPed>"
  BS_Result/3 -> ToWs_Result_Bus_Sig3/1  "<AccPed_facCompAcs>"
  BS_Result/4 -> ToWs_Result_Bus_Sig4/1  "<AccPed_trqComp>"
  BS_Result/5 -> ToWs_Result_Bus_Sig5/1  "<AccPed_stBrkDes>"
  BS_Result/6 -> ToWs_Result_Bus_Sig6/1  "<AccPed_stBrkDes_mp>"
  BS_Result/7 -> ToWs_Result_Bus_Sig7/1  "<AccPed_trqDifBrk_mp>"
  BS_Result/8 -> ToWs_Result_Bus_Sig8/1  "<AccPed_rBrk50_mp>"
  BS_Result/9 -> ToWs_Result_Bus_Sig9/1  "<AccPed_trqDesPull>"
  specifyOutputs/1(result) -> result/1

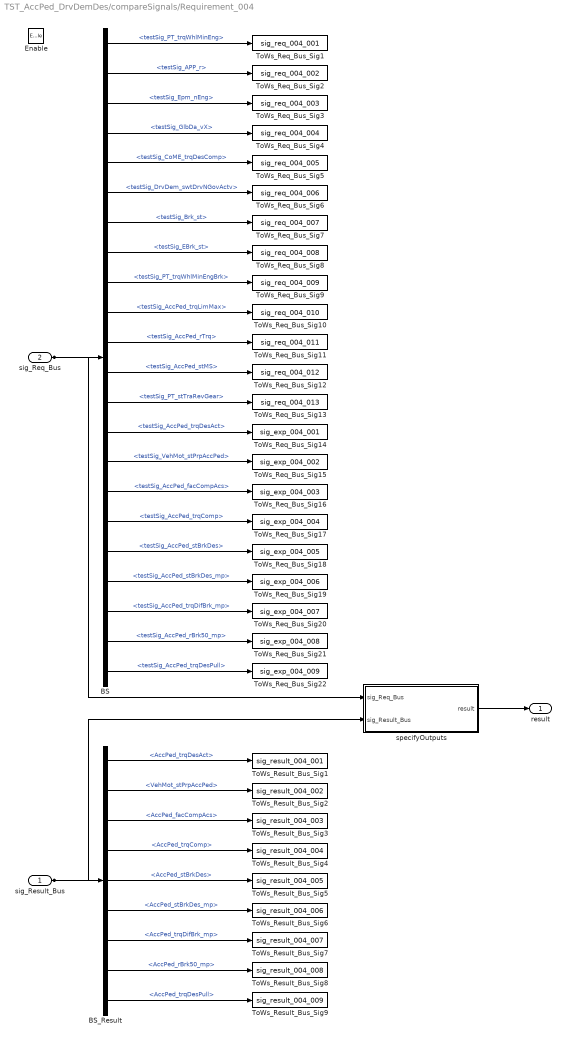
== system TST_AccPed_DrvDemDes/compareSignals/Requirement_004 ==
  sig_Result_Bus : Inport
  sig_Req_Bus : Inport  Port=2
  Enable : EnablePort
  BS : BusSelector  OutputSignals=testSig_PT_trqWhlMinEng,testSig_APP_r,testSig_Epm_nEng,testSig_GlbDa_vX,testSig_CoME_trqDesComp,testSig_DrvDem_swtDrvNGovActv,testSig_Brk_st,testSig_EBrk_st,testSig_PT_trqWhlMinEngBrk,testSig_AccPed_trqLimMax,testSig_AccPed_rTrq,testSig_AccPed_stMS,testSig_PT_stTraRevGear,testSig_AccPed_trqDesAct,testSig_VehMot_stPrpAccPed,testSig_AccPed_facCompAcs,testSig_AccPed_trqComp,testSig_AccPed_stBrkDes,testSig_AccPed_stBrkDes_mp,testSig_AccPed_trqDifBrk_mp,testSig_AccPed_rBrk50_mp,testSig_AccPed_trqDesPull
  BS_Result : BusSelector  OutputSignals=AccPed_trqDesAct,VehMot_stPrpAccPed,AccPed_facCompAcs,AccPed_trqComp,AccPed_stBrkDes,AccPed_stBrkDes_mp,AccPed_trqDifBrk_mp,AccPed_rBrk50_mp,AccPed_trqDesPull
  ToWs_Req_Bus_Sig1 : ToWorkspace  VariableName=sig_req_004_001  SaveFormat=Structure With Time
  ToWs_Req_Bus_Sig10 : ToWorkspace  VariableName=sig_req_004_010  SaveFormat=Structure With Time
  ToWs_Req_Bus_Sig11 : ToWorkspace  VariableName=sig_req_004_011  SaveFormat=Structure With Time
  ToWs_Req_Bus_Sig12 : ToWorkspace  VariableName=sig_req_004_012  SaveFormat=Structure With Time
  ToWs_Req_Bus_Sig13 : ToWorkspace  VariableName=sig_req_004_013  SaveFormat=Structure With Time
  ToWs_Req_Bus_Sig14 : ToWorkspace  VariableName=sig_exp_004_001  SaveFormat=Structure With Time
  ToWs_Req_Bus_Sig15 : ToWorkspace  VariableName=sig_exp_004_002  SaveFormat=Structure With Time
  ToWs_Req_Bus_Sig16 : ToWorkspace  VariableName=sig_exp_004_003  SaveFormat=Structure With Time
  ToWs_Req_Bus_Sig17 : ToWorkspace  VariableName=sig_exp_004_004  SaveFormat=Structure With Time
  ToWs_Req_Bus_Sig18 : ToWorkspace  VariableName=sig_exp_004_005  SaveFormat=Structure With Time
  ToWs_Req_Bus_Sig19 : ToWorkspace  VariableName=sig_exp_004_006  SaveFormat=Structure With Time
  ToWs_Req_Bus_Sig2 : ToWorkspace  VariableName=sig_req_004_002  SaveFormat=Structure With Time
  ToWs_Req_Bus_Sig20 : ToWorkspace  VariableName=sig_exp_004_007  SaveFormat=Structure With Time
  ToWs_Req_Bus_Sig21 : ToWorkspace  VariableName=sig_exp_004_008  SaveFormat=Structure With Time
  ToWs_Req_Bus_Sig22 : ToWorkspace  VariableName=sig_exp_004_009  SaveFormat=Structure With Time
  ToWs_Req_Bus_Sig3 : ToWorkspace  VariableName=sig_req_004_003  SaveFormat=Structure With Time
  ToWs_Req_Bus_Sig4 : ToWorkspace  VariableName=sig_req_004_004  SaveFormat=Structure With Time
  ToWs_Req_Bus_Sig5 : ToWorkspace  VariableName=sig_req_004_005  SaveFormat=Structure With Time
  ToWs_Req_Bus_Sig6 : ToWorkspace  VariableName=sig_req_004_006  SaveFormat=Structure With Time
  ToWs_Req_Bus_Sig7 : ToWorkspace  VariableName=sig_req_004_007  SaveFormat=Structure With Time
  ToWs_Req_Bus_Sig8 : ToWorkspace  VariableName=sig_req_004_008  SaveFormat=Structure With Time
  ToWs_Req_Bus_Sig9 : ToWorkspace  VariableName=sig_req_004_009  SaveFormat=Structure With Time
  ToWs_Result_Bus_Sig1 : ToWorkspace  VariableName=sig_result_004_001  SaveFormat=Structure With Time
  ToWs_Result_Bus_Sig2 : ToWorkspace  VariableName=sig_result_004_002  SaveFormat=Structure With Time
  ToWs_Result_Bus_Sig3 : ToWorkspace  VariableName=sig_result_004_003  SaveFormat=Structure With Time
  ToWs_Result_Bus_Sig4 : ToWorkspace  VariableName=sig_result_004_004  SaveFormat=Structure With Time
  ToWs_Result_Bus_Sig5 : ToWorkspace  VariableName=sig_result_004_005  SaveFormat=Structure With Time
  ToWs_Result_Bus_Sig6 : ToWorkspace  VariableName=sig_result_004_006  SaveFormat=Structure With Time
  ToWs_Result_Bus_Sig7 : ToWorkspace  VariableName=sig_result_004_007  SaveFormat=Structure With Time
  ToWs_Result_Bus_Sig8 : ToWorkspace  VariableName=sig_result_004_008  SaveFormat=Structure With Time
  ToWs_Result_Bus_Sig9 : ToWorkspace  VariableName=sig_result_004_009  SaveFormat=Structure With Time
  specifyOutputs : Subsystem
  result : Outport
  wires:
  sig_Req_Bus/1 -> BS/1, specifyOutputs/1(sig_Req_Bus)
  BS/1 -> ToWs_Req_Bus_Sig1/1  "<testSig_PT_trqWhlMinEng>"
  BS/2 -> ToWs_Req_Bus_Sig2/1  "<testSig_APP_r>"
  BS/3 -> ToWs_Req_Bus_Sig3/1  "<testSig_Epm_nEng>"
  BS/4 -> ToWs_Req_Bus_Sig4/1  "<testSig_GlbDa_vX>"
  BS/5 -> ToWs_Req_Bus_Sig5/1  "<testSig_CoME_trqDesComp>"
  BS/6 -> ToWs_Req_Bus_Sig6/1  "<testSig_DrvDem_swtDrvNGovActv>"
  BS/7 -> ToWs_Req_Bus_Sig7/1  "<testSig_Brk_st>"
  BS/8 -> ToWs_Req_Bus_Sig8/1  "<testSig_EBrk_st>"
  BS/9 -> ToWs_Req_Bus_Sig9/1  "<testSig_PT_trqWhlMinEngBrk>"
  BS/10 -> ToWs_Req_Bus_Sig10/1  "<testSig_AccPed_trqLimMax>"
  BS/11 -> ToWs_Req_Bus_Sig11/1  "<testSig_AccPed_rTrq>"
  BS/12 -> ToWs_Req_Bus_Sig12/1  "<testSig_AccPed_stMS>"
  BS/13 -> ToWs_Req_Bus_Sig13/1  "<testSig_PT_stTraRevGear>"
  BS/14 -> ToWs_Req_Bus_Sig14/1  "<testSig_AccPed_trqDesAct>"
  BS/15 -> ToWs_Req_Bus_Sig15/1  "<testSig_VehMot_stPrpAccPed>"
  BS/16 -> ToWs_Req_Bus_Sig16/1  "<testSig_AccPed_facCompAcs>"
  BS/17 -> ToWs_Req_Bus_Sig17/1  "<testSig_AccPed_trqComp>"
  BS/18 -> ToWs_Req_Bus_Sig18/1  "<testSig_AccPed_stBrkDes>"
  BS/19 -> ToWs_Req_Bus_Sig19/1  "<testSig_AccPed_stBrkDes_mp>"
  BS/20 -> ToWs_Req_Bus_Sig20/1  "<testSig_AccPed_trqDifBrk_mp>"
  BS/21 -> ToWs_Req_Bus_Sig21/1  "<testSig_AccPed_rBrk50_mp>"
  BS/22 -> ToWs_Req_Bus_Sig22/1  "<testSig_AccPed_trqDesPull>"
  sig_Result_Bus/1 -> BS_Result/1, specifyOutputs/2(sig_Result_Bus)
  BS_Result/1 -> ToWs_Result_Bus_Sig1/1  "<AccPed_trqDesAct>"
  BS_Result/2 -> ToWs_Result_Bus_Sig2/1  "<VehMot_stPrpAccPed>"
  BS_Result/3 -> ToWs_Result_Bus_Sig3/1  "<AccPed_facCompAcs>"
  BS_Result/4 -> ToWs_Result_Bus_Sig4/1  "<AccPed_trqComp>"
  BS_Result/5 -> ToWs_Result_Bus_Sig5/1  "<AccPed_stBrkDes>"
  BS_Result/6 -> ToWs_Result_Bus_Sig6/1  "<AccPed_stBrkDes_mp>"
  BS_Result/7 -> ToWs_Result_Bus_Sig7/1  "<AccPed_trqDifBrk_mp>"
  BS_Result/8 -> ToWs_Result_Bus_Sig8/1  "<AccPed_rBrk50_mp>"
  BS_Result/9 -> ToWs_Result_Bus_Sig9/1  "<AccPed_trqDesPull>"
  specifyOutputs/1(result) -> result/1

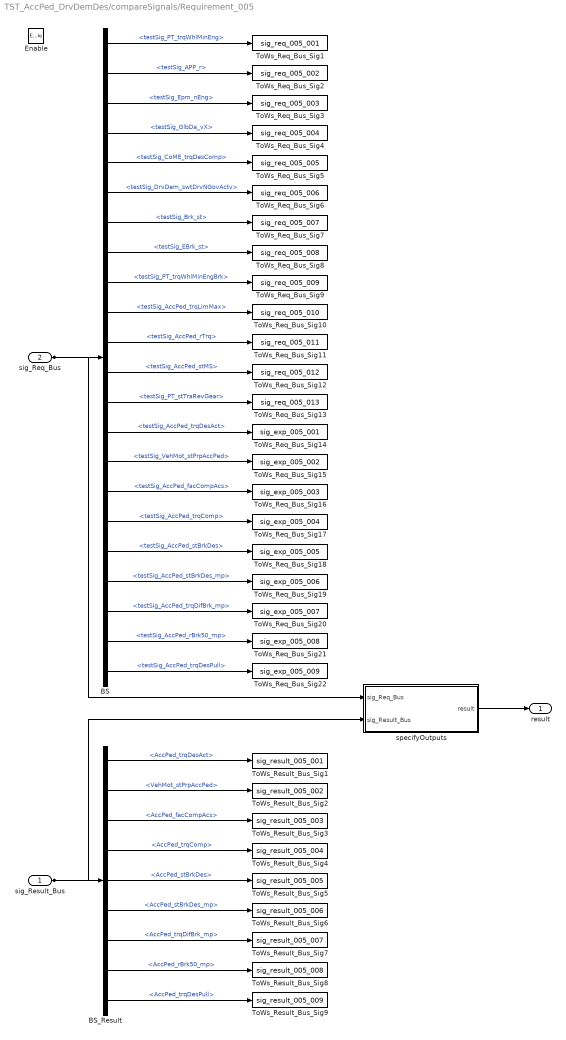
== system TST_AccPed_DrvDemDes/compareSignals/Requirement_005 ==
  sig_Result_Bus : Inport
  sig_Req_Bus : Inport  Port=2
  Enable : EnablePort
  BS : BusSelector  OutputSignals=testSig_PT_trqWhlMinEng,testSig_APP_r,testSig_Epm_nEng,testSig_GlbDa_vX,testSig_CoME_trqDesComp,testSig_DrvDem_swtDrvNGovActv,testSig_Brk_st,testSig_EBrk_st,testSig_PT_trqWhlMinEngBrk,testSig_AccPed_trqLimMax,testSig_AccPed_rTrq,testSig_AccPed_stMS,testSig_PT_stTraRevGear,testSig_AccPed_trqDesAct,testSig_VehMot_stPrpAccPed,testSig_AccPed_facCompAcs,testSig_AccPed_trqComp,testSig_AccPed_stBrkDes,testSig_AccPed_stBrkDes_mp,testSig_AccPed_trqDifBrk_mp,testSig_AccPed_rBrk50_mp,testSig_AccPed_trqDesPull
  BS_Result : BusSelector  OutputSignals=AccPed_trqDesAct,VehMot_stPrpAccPed,AccPed_facCompAcs,AccPed_trqComp,AccPed_stBrkDes,AccPed_stBrkDes_mp,AccPed_trqDifBrk_mp,AccPed_rBrk50_mp,AccPed_trqDesPull
  ToWs_Req_Bus_Sig1 : ToWorkspace  VariableName=sig_req_005_001  SaveFormat=Structure With Time
  ToWs_Req_Bus_Sig10 : ToWorkspace  VariableName=sig_req_005_010  SaveFormat=Structure With Time
  ToWs_Req_Bus_Sig11 : ToWorkspace  VariableName=sig_req_005_011  SaveFormat=Structure With Time
  ToWs_Req_Bus_Sig12 : ToWorkspace  VariableName=sig_req_005_012  SaveFormat=Structure With Time
  ToWs_Req_Bus_Sig13 : ToWorkspace  VariableName=sig_req_005_013  SaveFormat=Structure With Time
  ToWs_Req_Bus_Sig14 : ToWorkspace  VariableName=sig_exp_005_001  SaveFormat=Structure With Time
  ToWs_Req_Bus_Sig15 : ToWorkspace  VariableName=sig_exp_005_002  SaveFormat=Structure With Time
  ToWs_Req_Bus_Sig16 : ToWorkspace  VariableName=sig_exp_005_003  SaveFormat=Structure With Time
  ToWs_Req_Bus_Sig17 : ToWorkspace  VariableName=sig_exp_005_004  SaveFormat=Structure With Time
  ToWs_Req_Bus_Sig18 : ToWorkspace  VariableName=sig_exp_005_005  SaveFormat=Structure With Time
  ToWs_Req_Bus_Sig19 : ToWorkspace  VariableName=sig_exp_005_006  SaveFormat=Structure With Time
  ToWs_Req_Bus_Sig2 : ToWorkspace  VariableName=sig_req_005_002  SaveFormat=Structure With Time
  ToWs_Req_Bus_Sig20 : ToWorkspace  VariableName=sig_exp_005_007  SaveFormat=Structure With Time
  ToWs_Req_Bus_Sig21 : ToWorkspace  VariableName=sig_exp_005_008  SaveFormat=Structure With Time
  ToWs_Req_Bus_Sig22 : ToWorkspace  VariableName=sig_exp_005_009  SaveFormat=Structure With Time
  ToWs_Req_Bus_Sig3 : ToWorkspace  VariableName=sig_req_005_003  SaveFormat=Structure With Time
  ToWs_Req_Bus_Sig4 : ToWorkspace  VariableName=sig_req_005_004  SaveFormat=Structure With Time
  ToWs_Req_Bus_Sig5 : ToWorkspace  VariableName=sig_req_005_005  SaveFormat=Structure With Time
  ToWs_Req_Bus_Sig6 : ToWorkspace  VariableName=sig_req_005_006  SaveFormat=Structure With Time
  ToWs_Req_Bus_Sig7 : ToWorkspace  VariableName=sig_req_005_007  SaveFormat=Structure With Time
  ToWs_Req_Bus_Sig8 : ToWorkspace  VariableName=sig_req_005_008  SaveFormat=Structure With Time
  ToWs_Req_Bus_Sig9 : ToWorkspace  VariableName=sig_req_005_009  SaveFormat=Structure With Time
  ToWs_Result_Bus_Sig1 : ToWorkspace  VariableName=sig_result_005_001  SaveFormat=Structure With Time
  ToWs_Result_Bus_Sig2 : ToWorkspace  VariableName=sig_result_005_002  SaveFormat=Structure With Time
  ToWs_Result_Bus_Sig3 : ToWorkspace  VariableName=sig_result_005_003  SaveFormat=Structure With Time
  ToWs_Result_Bus_Sig4 : ToWorkspace  VariableName=sig_result_005_004  SaveFormat=Structure With Time
  ToWs_Result_Bus_Sig5 : ToWorkspace  VariableName=sig_result_005_005  SaveFormat=Structure With Time
  ToWs_Result_Bus_Sig6 : ToWorkspace  VariableName=sig_result_005_006  SaveFormat=Structure With Time
  ToWs_Result_Bus_Sig7 : ToWorkspace  VariableName=sig_result_005_007  SaveFormat=Structure With Time
  ToWs_Result_Bus_Sig8 : ToWorkspace  VariableName=sig_result_005_008  SaveFormat=Structure With Time
  ToWs_Result_Bus_Sig9 : ToWorkspace  VariableName=sig_result_005_009  SaveFormat=Structure With Time
  specifyOutputs : Subsystem
  result : Outport
  wires:
  sig_Req_Bus/1 -> BS/1, specifyOutputs/1(sig_Req_Bus)
  BS/1 -> ToWs_Req_Bus_Sig1/1  "<testSig_PT_trqWhlMinEng>"
  BS/2 -> ToWs_Req_Bus_Sig2/1  "<testSig_APP_r>"
  BS/3 -> ToWs_Req_Bus_Sig3/1  "<testSig_Epm_nEng>"
  BS/4 -> ToWs_Req_Bus_Sig4/1  "<testSig_GlbDa_vX>"
  BS/5 -> ToWs_Req_Bus_Sig5/1  "<testSig_CoME_trqDesComp>"
  BS/6 -> ToWs_Req_Bus_Sig6/1  "<testSig_DrvDem_swtDrvNGovActv>"
  BS/7 -> ToWs_Req_Bus_Sig7/1  "<testSig_Brk_st>"
  BS/8 -> ToWs_Req_Bus_Sig8/1  "<testSig_EBrk_st>"
  BS/9 -> ToWs_Req_Bus_Sig9/1  "<testSig_PT_trqWhlMinEngBrk>"
  BS/10 -> ToWs_Req_Bus_Sig10/1  "<testSig_AccPed_trqLimMax>"
  BS/11 -> ToWs_Req_Bus_Sig11/1  "<testSig_AccPed_rTrq>"
  BS/12 -> ToWs_Req_Bus_Sig12/1  "<testSig_AccPed_stMS>"
  BS/13 -> ToWs_Req_Bus_Sig13/1  "<testSig_PT_stTraRevGear>"
  BS/14 -> ToWs_Req_Bus_Sig14/1  "<testSig_AccPed_trqDesAct>"
  BS/15 -> ToWs_Req_Bus_Sig15/1  "<testSig_VehMot_stPrpAccPed>"
  BS/16 -> ToWs_Req_Bus_Sig16/1  "<testSig_AccPed_facCompAcs>"
  BS/17 -> ToWs_Req_Bus_Sig17/1  "<testSig_AccPed_trqComp>"
  BS/18 -> ToWs_Req_Bus_Sig18/1  "<testSig_AccPed_stBrkDes>"
  BS/19 -> ToWs_Req_Bus_Sig19/1  "<testSig_AccPed_stBrkDes_mp>"
  BS/20 -> ToWs_Req_Bus_Sig20/1  "<testSig_AccPed_trqDifBrk_mp>"
  BS/21 -> ToWs_Req_Bus_Sig21/1  "<testSig_AccPed_rBrk50_mp>"
  BS/22 -> ToWs_Req_Bus_Sig22/1  "<testSig_AccPed_trqDesPull>"
  sig_Result_Bus/1 -> BS_Result/1, specifyOutputs/2(sig_Result_Bus)
  BS_Result/1 -> ToWs_Result_Bus_Sig1/1  "<AccPed_trqDesAct>"
  BS_Result/2 -> ToWs_Result_Bus_Sig2/1  "<VehMot_stPrpAccPed>"
  BS_Result/3 -> ToWs_Result_Bus_Sig3/1  "<AccPed_facCompAcs>"
  BS_Result/4 -> ToWs_Result_Bus_Sig4/1  "<AccPed_trqComp>"
  BS_Result/5 -> ToWs_Result_Bus_Sig5/1  "<AccPed_stBrkDes>"
  BS_Result/6 -> ToWs_Result_Bus_Sig6/1  "<AccPed_stBrkDes_mp>"
  BS_Result/7 -> ToWs_Result_Bus_Sig7/1  "<AccPed_trqDifBrk_mp>"
  BS_Result/8 -> ToWs_Result_Bus_Sig8/1  "<AccPed_rBrk50_mp>"
  BS_Result/9 -> ToWs_Result_Bus_Sig9/1  "<AccPed_trqDesPull>"
  specifyOutputs/1(result) -> result/1

== system TST_AccPed_DrvDemDes/compareSignals/Requirement_006 ==
  sig_Result_Bus : Inport
  sig_Req_Bus : Inport  Port=2
  Enable : EnablePort
  BS : BusSelector  OutputSignals=testSig_PT_trqWhlMinEng,testSig_APP_r,testSig_Epm_nEng,testSig_GlbDa_vX,testSig_CoME_trqDesComp,testSig_DrvDem_swtDrvNGovActv,testSig_Brk_st,testSig_EBrk_st,testSig_PT_trqWhlMinEngBrk,testSig_AccPed_trqLimMax,testSig_AccPed_rTrq,testSig_AccPed_stMS,testSig_PT_stTraRevGear,testSig_AccPed_trqDesAct,testSig_VehMot_stPrpAccPed,testSig_AccPed_facCompAcs,testSig_AccPed_trqComp,testSig_AccPed_stBrkDes,testSig_AccPed_stBrkDes_mp,testSig_AccPed_trqDifBrk_mp,testSig_AccPed_rBrk50_mp,testSig_AccPed_trqDesPull
  BS_Result : BusSelector  OutputSignals=AccPed_trqDesAct,VehMot_stPrpAccPed,AccPed_facCompAcs,AccPed_trqComp,AccPed_stBrkDes,AccPed_stBrkDes_mp,AccPed_trqDifBrk_mp,AccPed_rBrk50_mp,AccPed_trqDesPull
  ToWs_Req_Bus_Sig1 : ToWorkspace  VariableName=sig_req_006_001  SaveFormat=Structure With Time
  ToWs_Req_Bus_Sig10 : ToWorkspace  VariableName=sig_req_006_010  SaveFormat=Structure With Time
  ToWs_Req_Bus_Sig11 : ToWorkspace  VariableName=sig_req_006_011  SaveFormat=Structure With Time
  ToWs_Req_Bus_Sig12 : ToWorkspace  VariableName=sig_req_006_012  SaveFormat=Structure With Time
  ToWs_Req_Bus_Sig13 : ToWorkspace  VariableName=sig_req_006_013  SaveFormat=Structure With Time
  ToWs_Req_Bus_Sig14 : ToWorkspace  VariableName=sig_exp_006_001  SaveFormat=Structure With Time
  ToWs_Req_Bus_Sig15 : ToWorkspace  VariableName=sig_exp_006_002  SaveFormat=Structure With Time
  ToWs_Req_Bus_Sig16 : ToWorkspace  VariableName=sig_exp_006_003  SaveFormat=Structure With Time
  ToWs_Req_Bus_Sig17 : ToWorkspace  VariableName=sig_exp_006_004  SaveFormat=Structure With Time
  ToWs_Req_Bus_Sig18 : ToWorkspace  VariableName=sig_exp_006_005  SaveFormat=Structure With Time
  ToWs_Req_Bus_Sig19 : ToWorkspace  VariableName=sig_exp_006_006  SaveFormat=Structure With Time
  ToWs_Req_Bus_Sig2 : ToWorkspace  VariableName=sig_req_006_002  SaveFormat=Structure With Time
  ToWs_Req_Bus_Sig20 : ToWorkspace  VariableName=sig_exp_006_007  SaveFormat=Structure With Time
  ToWs_Req_Bus_Sig21 : ToWorkspace  VariableName=sig_exp_006_008  SaveFormat=Structure With Time
  ToWs_Req_Bus_Sig22 : ToWorkspace  VariableName=sig_exp_006_009  SaveFormat=Structure With Time
  ToWs_Req_Bus_Sig3 : ToWorkspace  VariableName=sig_req_006_003  SaveFormat=Structure With Time
  ToWs_Req_Bus_Sig4 : ToWorkspace  VariableName=sig_req_006_004  SaveFormat=Structure With Time
  ToWs_Req_Bus_Sig5 : ToWorkspace  VariableName=sig_req_006_005  SaveFormat=Structure With Time
  ToWs_Req_Bus_Sig6 : ToWorkspace  VariableName=sig_req_006_006  SaveFormat=Structure With Time
  ToWs_Req_Bus_Sig7 : ToWorkspace  VariableName=sig_req_006_007  SaveFormat=Structure With Time
  ToWs_Req_Bus_Sig8 : ToWorkspace  VariableName=sig_req_006_008  SaveFormat=Structure With Time
  ToWs_Req_Bus_Sig9 : ToWorkspace  VariableName=sig_req_006_009  SaveFormat=Structure With Time
  ToWs_Result_Bus_Sig1 : ToWorkspace  VariableName=sig_result_006_001  SaveFormat=Structure With Time
  ToWs_Result_Bus_Sig2 : ToWorkspace  VariableName=sig_result_006_002  SaveFormat=Structure With Time
  ToWs_Result_Bus_Sig3 : ToWorkspace  VariableName=sig_result_006_003  SaveFormat=Structure With Time
  ToWs_Result_Bus_Sig4 : ToWorkspace  VariableName=sig_result_006_004  SaveFormat=Structure With Time
  ToWs_Result_Bus_Sig5 : ToWorkspace  VariableName=sig_result_006_005  SaveFormat=Structure With Time
  ToWs_Result_Bus_Sig6 : ToWorkspace  VariableName=sig_result_006_006  SaveFormat=Structure With Time
  ToWs_Result_Bus_Sig7 : ToWorkspace  VariableName=sig_result_006_007  SaveFormat=Structure With Time
  ToWs_Result_Bus_Sig8 : ToWorkspace  VariableName=sig_result_006_008  SaveFormat=Structure With Time
  ToWs_Result_Bus_Sig9 : ToWorkspace  VariableName=sig_result_006_009  SaveFormat=Structure With Time
  specifyOutputs : Subsystem
  result : Outport
  wires:
  sig_Req_Bus/1 -> BS/1, specifyOutputs/1(sig_Req_Bus)
  BS/1 -> ToWs_Req_Bus_Sig1/1  "<testSig_PT_trqWhlMinEng>"
  BS/2 -> ToWs_Req_Bus_Sig2/1  "<testSig_APP_r>"
  BS/3 -> ToWs_Req_Bus_Sig3/1  "<testSig_Epm_nEng>"
  BS/4 -> ToWs_Req_Bus_Sig4/1  "<testSig_GlbDa_vX>"
  BS/5 -> ToWs_Req_Bus_Sig5/1  "<testSig_CoME_trqDesComp>"
  BS/6 -> ToWs_Req_Bus_Sig6/1  "<testSig_DrvDem_swtDrvNGovActv>"
  BS/7 -> ToWs_Req_Bus_Sig7/1  "<testSig_Brk_st>"
  BS/8 -> ToWs_Req_Bus_Sig8/1  "<testSig_EBrk_st>"
  BS/9 -> ToWs_Req_Bus_Sig9/1  "<testSig_PT_trqWhlMinEngBrk>"
  BS/10 -> ToWs_Req_Bus_Sig10/1  "<testSig_AccPed_trqLimMax>"
  BS/11 -> ToWs_Req_Bus_Sig11/1  "<testSig_AccPed_rTrq>"
  BS/12 -> ToWs_Req_Bus_Sig12/1  "<testSig_AccPed_stMS>"
  BS/13 -> ToWs_Req_Bus_Sig13/1  "<testSig_PT_stTraRevGear>"
  BS/14 -> ToWs_Req_Bus_Sig14/1  "<testSig_AccPed_trqDesAct>"
  BS/15 -> ToWs_Req_Bus_Sig15/1  "<testSig_VehMot_stPrpAccPed>"
  BS/16 -> ToWs_Req_Bus_Sig16/1  "<testSig_AccPed_facCompAcs>"
  BS/17 -> ToWs_Req_Bus_Sig17/1  "<testSig_AccPed_trqComp>"
  BS/18 -> ToWs_Req_Bus_Sig18/1  "<testSig_AccPed_stBrkDes>"
  BS/19 -> ToWs_Req_Bus_Sig19/1  "<testSig_AccPed_stBrkDes_mp>"
  BS/20 -> ToWs_Req_Bus_Sig20/1  "<testSig_AccPed_trqDifBrk_mp>"
  BS/21 -> ToWs_Req_Bus_Sig21/1  "<testSig_AccPed_rBrk50_mp>"
  BS/22 -> ToWs_Req_Bus_Sig22/1  "<testSig_AccPed_trqDesPull>"
  sig_Result_Bus/1 -> BS_Result/1, specifyOutputs/2(sig_Result_Bus)
  BS_Result/1 -> ToWs_Result_Bus_Sig1/1  "<AccPed_trqDesAct>"
  BS_Result/2 -> ToWs_Result_Bus_Sig2/1  "<VehMot_stPrpAccPed>"
  BS_Result/3 -> ToWs_Result_Bus_Sig3/1  "<AccPed_facCompAcs>"
  BS_Result/4 -> ToWs_Result_Bus_Sig4/1  "<AccPed_trqComp>"
  BS_Result/5 -> ToWs_Result_Bus_Sig5/1  "<AccPed_stBrkDes>"
  BS_Result/6 -> ToWs_Result_Bus_Sig6/1  "<AccPed_stBrkDes_mp>"
  BS_Result/7 -> ToWs_Result_Bus_Sig7/1  "<AccPed_trqDifBrk_mp>"
  BS_Result/8 -> ToWs_Result_Bus_Sig8/1  "<AccPed_rBrk50_mp>"
  BS_Result/9 -> ToWs_Result_Bus_Sig9/1  "<AccPed_trqDesPull>"
  specifyOutputs/1(result) -> result/1
